simulink library "S2_aero_lib"  (Simulink 6.6)
libraries: simulink x1
settings Model: Creator=amurch  LastModifiedBy=Austin Murch

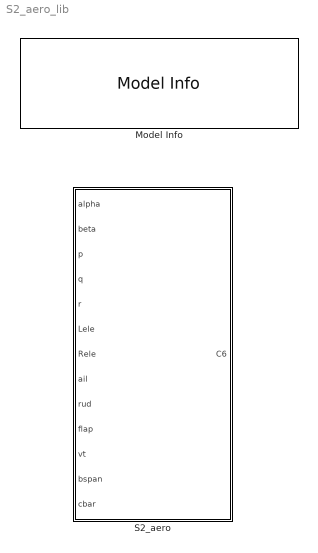
== system S2_aero_lib ==
  Model Info : simulink/Model-Wide Utilities/Model Info  SystemSampleTime=-1  InitialBlockCM=None  BlockCM=None  Frame=on  DisplayStringWithTags=|  HorizontalTextAlignment=Center  LeftAlignmentValue=0.5  SourceBlockDiagram=S2_aero_lib  TagMaxNumber=20
      | S2 Aerodynamic Model Library
      | %<ModelVersion>
      | Last modified by %<LastModifiedBy> on %<LastModificationDate>
  S2_aero : Stateflow chart

== matlab function S2_aero ==
  data: alpha input inherited; C6 output inherited; beta input inherited; p input inherited; q input inherited; r input inherited; Lele input inherited; Rele input inherited; ail input inherited; rud input inherited; flap input inherited; vt input inherited; bspan input inherited; cbar input inherited
function C6 =s2_aero(alpha,beta,p,q,r,Lele,Rele,ail,rud,flap,vt,bspan,cbar)
%
%  S2_AERO  Computes non-dimensional aerodynamic coefficients for the S2 aircraft.
%
%  Usage:
%  [C6]=s2_aero(alpha,beta,phat,qhat,rhat,throttle,ele,ail,rud,flap);
%
%  Description:
%
%    Computes the non-dimensional aerodynamic force and moment
%    coefficients for the S2 single-engine L-1011 model aircraft 
%    using frequency separation modeling and flight data from 
%    deployment 2007.02, September 2007.  
%
%
%  Input:
%    
%     alpha = angle of attack, deg.
%      beta = sideslip angle, deg.
%      phat = nondimensional roll rate (pb/2V), rad/sec.
%      qhat = nondimensional pitch rate (qc/2V), rad/sec.
%      rhat = nondimensional yaw rate (rb/2V), rad/sec.
%      Lele = left elevator deflection, deg.
%      Rele = right elevator deflection, deg.
%       ail = aileron deflection, deg.
%       rud = rudder deflection, deg.
%      flap = flap deflections, deg.
%        c = constants.
%            c.lim   = array of hard limits for the controls.

%  Output:
%
%     CX = body axis x force coefficient.
%     CY = body axis y force coefficient.
%     CZ = body axis z force coefficient.
%     C1 = rolling moment coefficient.
%     Cm = pitching moment coefficient.
%     Cn = yawing moment coefficient.
%

%
%    Calls:
%      s2_xo.m, s2_zo.m, s2_mo.m
%      s2_xd.m, s2_zd.m, s2_md.m
%      s2_yo.m, s2_1o.m, s2_no.m
%      s2_yd.m, s2_1d.m, s2_nd.m
%
%    Author:  Eugene A. Morelli
%
%    History:  
%      18 Feb 2008 - Created and debugged, EAM.
%      13 May 2008 - Modified for use in Simulink, AMM.
%
%  Copyright (C) 2008  Eugene A. Morelli
%
%  This program carries no warranty, not even the implied 
%  warranty of merchantability or fitness for a particular purpose.  
%
%  Please email bug reports or suggestions for improvements to:
%
%      e.a.morelli@nasa.gov
%
c.lim = [0 100;-30 30;-20 20;-30 30;0 30];
dtr=pi/180;
betar=beta*dtr;
alphar=alpha*dtr;
Lelr=Lele*dtr;
Relr=Rele*dtr;
elr = 0.5*(Lelr + Relr);
ailr=ail*dtr;
rdrr=rud*dtr;
flpr=flap*dtr;
phat = p*bspan/(2*vt);
qhat = q*cbar/(2*vt);
rhat = r*bspan/(2*vt);
ele_loc =10/12; % ft, location of center of elevator relative to butt line (approx)

%
%  Get the base terms.  
%
CXo=s2_xo(alphar,elr,flpr,c);
CZo=s2_zo(alphar,elr,flpr,c);
Cmo=s2_mo(alphar,elr,flpr,c);
%
CYo=s2_yo(alphar,elr,flpr,c);
C1o=s2_1o(alphar,elr,flpr,c);
Cno=s2_no(alphar,elr,flpr,c);
%
%  Get the stability and control derivatives. 
%
[CXa,CXq,CXel,CXflp]=s2_xd(alphar,elr,flpr,c);
[CZa,CZq,CZel,CZflp]=s2_zd(alphar,elr,flpr,c);
[Cma,Cmq,Cmel,Cmflp]=s2_md(alphar,elr,flpr,c);
%
[CYb,CYp,CYr,CYail,CYrdr]=s2_yd(alphar,elr,flpr,c);
[C1b,C1p,C1r,C1ail,C1rdr]=s2_1d(alphar,elr,flpr,c);
[Cnb,Cnp,Cnr,Cnail,Cnrdr]=s2_nd(alphar,elr,flpr,c);
%
%  Assemble the force and moment coefficients.
%
CX = CXo + CXq*qhat + CXflp*flpr + CXel*(Lelr + Relr)/2;
CZ = CZo + CZq*qhat + CZflp*flpr + CZel*(Lelr + Relr)/2;
Cm = Cmo + Cmq*qhat + Cmflp*flpr + Cmel*(Lelr + Relr)/2;
%
CY = CYo + CYb*betar + CYp*phat + CYr*rhat + CYail*ailr + CYrdr*rdrr;
C1 = C1o + C1b*betar + C1p*phat + C1r*rhat + C1ail*ailr + C1rdr*rdrr + CZel*ele_loc*(Relr - Lelr)/2/bspan;
Cn = Cno + Cnb*betar + Cnp*phat + Cnr*rhat + Cnail*ailr + Cnrdr*rdrr + CXel*ele_loc*(Lelr - Relr)/2/bspan;
%
% Apply some sanity limits to the coefficients
%
C6 = max(min([CX CY CZ C1 Cm Cn],[3 2 4 2 4 4]),-[3 2 4 2 4 4]);

function [CXo] = s2_xo(alpha,el,flp,c)
%
%  S2_XO  Computes the CX base aerodynamics.
%
%  Usage: CXo = s2_xo(alpha,el,flp,c);
%
%  Description:
%
%    Computes the CX base aerodynamics
%    for the S2 single-engine L-1011 model
%    aircraft nonlinear simulation.  
%
%  Input:
%    
%     alpha = angle of attack, rad.
%        el = elevator deflection, rad.
%       flp = flap deflection, rad.
%         c = c.c(1) through c.c(9) = inertia constants.
%  Output:
%
%       CXo = CX base aerodynamic term. 
%

%
%    Calls:
%      comfun.m
%
%    Author:  Eugene A. Morelli
%
%    History:  
%      05 May  2008 - Created and debugged, EAM.
%
%  Copyright (C) 2008  Eugene A. Morelli
%
%  This program carries no warranty, not even the implied 
%  warranty of merchantability or fitness for a particular purpose.  
%
%  Please email bug reports or suggestions for improvements to:
%
%      e.a.morelli@nasa.gov
%
dtr=pi/180;
x=[alpha,min(0,alpha-15*dtr)];
%
%  Cruise, flaps up, gear up, from flt9, man6.  
%
% IPXo=[0,1,11,10]';
% PXo=[ -0.080800885759421;...
%        0.820366736327515;...
%      -10.010727396895621;...
%        3.057073727021578];
% IPXo=[1,0,11,10]';
% PXo=[  0.822422596042795
%       -0.089099684117894
%      -11.674020983809706
%        3.480804446726977];
IPXo=[1,0,4,3]';
PXo=[  0.384250553871670;...
      -0.055695436673931;...
     -38.087897257727697;...
      14.888723078459181];
% IPXo=[0,1,2]';
% PXo=[ -0.070197931596795;...
%        0.703156250629286;...
%        0.250092538873889];
CXo=comfun(x,PXo,IPXo);
%
%  Approach, flaps down, gear down, from flt9, man9.
%
IPXoa=[0,1,2,11]';
PXoa=[ -0.341975568896875;...
        2.311938939310571;...
       -2.634264867496561;...
       -3.328376671167995];
CXoa=comfun(x,PXoa,IPXoa);
%
%  Compute df = fraction of full flap deflection.  
%
df=max(c.lim(5,1),min(flp/dtr,c.lim(5,2)))/c.lim(5,2);
%
%  Schedule linearly based on flap deflection.
%
CXo=CXo + df*(CXoa-CXo);
return


function [CXa,CXq,CXel,CXflp] = s2_xd(alpha,el,flp,c)
%
%  S2_XD  Computes the CX stability and control derivatives.
%
%  Usage: [CXa,CXq,CXel,CXflp] = s2_xd(alpha,el,flp,c);
%
%  Description:
%
%    Computes the CX stability and control derivatives 
%    for the S2 single-engine L-1011 model
%    aircraft nonlinear simulation.  
%
%  Input:
%    
%     alpha = angle of attack, rad.
%        el = elevator deflection, rad.
%       flp = flap deflection, rad.
%         c = c.c(1) through c.c(9) = inertia constants.
%  Output:
%
%       CXa = CX stability derivative for angle of attack, 1/rad.  
%       CXq = CX stability derivative for non-dimensional pitch rate.
%      CXel = CX control derivative for elevator deflection, 1/rad.
%     CXflp = CX control derivative for flap deflection, 1/rad.
%

%
%    Calls:
%      None
%
%    Author:  Eugene A. Morelli
%
%    History:  
%      05 May  2008 - Created and debugged, EAM.
%
%  Copyright (C) 2008  Eugene A. Morelli
%
%  This program carries no warranty, not even the implied 
%  warranty of merchantability or fitness for a particular purpose.  
%
%  Please email bug reports or suggestions for improvements to:
%
%      e.a.morelli@nasa.gov
%

%
%  Cruise, flaps up, gear up, from flt13, man8a.
%
CXa=0.4215;
CXq=0;
CXel=0.0375;
CXflp=0;
%
%  Approach, full flaps, gear down, from flt12, man6.
%
CXaa=0.4008;
CXqa=0;
CXela=0.0216;
CXflpa=0;
%
%  Compute df = fraction of full flap deflection.  
%
df=max(c.lim(5,1),min(flp*180/pi,c.lim(5,2)))/c.lim(5,2);
%
%  Schedule linearly based on flap deflection.
%
CXa=CXa + df*(CXaa-CXa);
CXq=CXq + df*(CXqa-CXq);
CXel=CXel + df*(CXela-CXel);
CXflp=CXflp + df*(CXflpa-CXflp);
return

function CYo = s2_yo(alpha,el,flp,c)
%
%  S2_YO  Computes the CY base aerodynamics.
%
%  Usage: CYo = s2_yo(alpha,el,flp,c);
%
%  Description:
%
%    Computes the CY base aerodynamics
%    for the S2 single-engine L-1011 model
%    aircraft nonlinear simulation.  
%
%  Input:
%    
%     alpha = angle of attack, rad.
%        el = elevator deflection, rad.
%       flp = flap deflection, rad.
%         c = c.c(1) through c.c(9) = inertia constants.
%  Output:
%
%       CYo = CY base aerodynamic term. 
%

%
%    Calls:
%      None
%
%    Author:  Eugene A. Morelli
%
%    History:  
%      05 May  2008 - Created and debugged, EAM.
%
%  Copyright (C) 2008  Eugene A. Morelli
%
%  This program carries no warranty, not even the implied 
%  warranty of merchantability or fitness for a particular purpose.  
%
%  Please email bug reports or suggestions for improvements to:
%
%      e.a.morelli@nasa.gov
%

CYo=0;
return

function [CYb,CYp,CYr,CYail,CYrdr] = s2_yd(alpha,el,flp,c)
%
%  S2_YD  Computes the CY stability and control derivatives.
%
%  Usage: [CYb,CYp,CYr,CYail,CYrdr] = s2_yd(alpha,el,flp,c);
%
%  Description:
%
%    Computes the CY stability and control derivatives 
%    for the S2 single-engine L-1011 model
%    aircraft nonlinear simulation.  
%
%  Input:
%    
%     alpha = angle of attack, rad.
%        el = elevator deflection, rad.
%       flp = flap deflection, rad.
%         c = c.c(1) through c.c(9) = inertia constants.
%             c.mass  = aircraft mass, slugs.
%             c.xcg   = longitudinal (MS) CG location, percent MAC.
%             c.ycg   = lateral (BL) CG location, in.
%             c.zcg   = vertical (WL) CG location, in.
%             c.xcgr  = reference longitudinal (MS) CG location, percent MAC.
%             c.heng  = angular momentum for rotating mass of the propulsion system.
%             c.sarea = wing reference area, ft2.
%             c.bspan = wing span, ft.
%             c.cbar  = wing MAC, ft.
%             c.lim   = array of hard limits for the controls.
%             c.ac    = name of the aircraft.
%             c.xfree = vector indicating free states for trim:
%                       = 1 for free state
%                       = 0 for fixed state
%             c.xinit = initial state vector for trim, 
%                       including fixed state values.
%             c.ufree = vector indicating free controls for trim:
%                       = 1 for free control
%                       = 0 for fixed control
%             c.uinit = initial control vector for trim, 
%                       including fixed control values.
%             c.gam   = flight path angle at trim, deg.
%             c.trate = turn rate at trim, deg/sec.
%             c.ltl   = trim or linearize flag
%                       =  1 for trim or steady condition
%                       =  0 for normal operation
%                       = -1 for linearization
%              c.ltrl = trim or linearize flag:
%                       = -1 for trim or steady condition
%                       =  0 for normal operation
%                       =  1 for linearization
%              c.lfi  = filter initialization flag:
%                       =  1 to initialize the filter
%                       =  0 for normal operation
%                       = -1 to skip the filtering (for numerical integration steps)
%              c.dt   = time step, sec.
%              c.x0   = initial state vector.
%              c.u0   = initial control vector.
%
%  Output:
%
%       CYb = CY stability derivative for angle of sideslip, 1/rad.  
%       CYp = CY stability derivative for non-dimensional roll rate.
%       CYr = CY stability derivative for non-dimensional yaw rate.
%     CYail = CY control derivative for aileron deflection, 1/rad.
%     CYrdr = CY control derivative for rudder deflection, 1/rad.
%

%
%    Calls:
%      None
%
%    Author:  Eugene A. Morelli
%
%    History:  
%      05 May  2008 - Created and debugged, EAM.
%
%  Copyright (C) 2008  Eugene A. Morelli
%
%  This program carries no warranty, not even the implied 
%  warranty of merchantability or fitness for a particular purpose.  
%
%  Please email bug reports or suggestions for improvements to:
%
%      e.a.morelli@nasa.gov
%

%
%  Cruise, flaps up, gear up, from flt13, man8a.
%
CYb=-0.7891;
CYp=0;
CYr=0;
CYail=0;
CYrdr=0.1881;
%
%  Approach, full flaps, gear down, from flt12, man6.
%
CYba=-1.0235;
CYpa=0;
CYra=0;
CYaila=0;
CYrdra=0.0835;
%
%  Compute df = fraction of full flap deflection.  
%
df=max(c.lim(5,1),min(flp*180/pi,c.lim(5,2)))/c.lim(5,2);
%
%  Schedule linearly based on flap deflection.
%
CYb=CYb + df*(CYba-CYb);
CYp=CYp + df*(CYpa-CYp);
CYr=CYr + df*(CYra-CYr);
CYail=CYail + df*(CYaila-CYail);
CYrdr=CYrdr + df*(CYrdra-CYrdr);
return


function CZo = s2_zo(alpha,el,flp,c)
%
%  S2_ZO  Computes the CZ base aerodynamics.
%
%  Usage: CZo = s2_zo(alpha,el,flp,c);
%
%  Description:
%
%    Computes the CZ base aerodynamics
%    for the S2 single-engine L-1011 model
%    aircraft nonlinear simulation.  
%
%  Input:
%    
%     alpha = angle of attack, rad.
%        el = elevator deflection, rad.
%       flp = flap deflection, rad.
%         c = c.c(1) through c.c(9) = inertia constants.
%             c.mass  = aircraft mass, slugs.
%             c.xcg   = longitudinal (MS) CG location, percent MAC.
%             c.ycg   = lateral (BL) CG location, in.
%             c.zcg   = vertical (WL) CG location, in.
%             c.xcgr  = reference longitudinal (MS) CG location, percent MAC.
%             c.heng  = angular momentum for rotating mass of the propulsion system.
%             c.sarea = wing reference area, ft2.
%             c.bspan = wing span, ft.
%             c.cbar  = wing MAC, ft.
%             c.lim   = array of hard limits for the controls.
%             c.ac    = name of the aircraft.
%             c.xfree = vector indicating free states for trim:
%                       = 1 for free state
%                       = 0 for fixed state
%             c.xinit = initial state vector for trim, 
%                       including fixed state values.
%             c.ufree = vector indicating free controls for trim:
%                       = 1 for free control
%                       = 0 for fixed control
%             c.uinit = initial control vector for trim, 
%                       including fixed control values.
%             c.gam   = flight path angle at trim, deg.
%             c.trate = turn rate at trim, deg/sec.
%             c.ltl   = trim or linearize flag
%                       =  1 for trim or steady condition
%                       =  0 for normal operation
%                       = -1 for linearization
%              c.ltrl = trim or linearize flag:
%                       = -1 for trim or steady condition
%                       =  0 for normal operation
%                       =  1 for linearization
%              c.lfi  = filter initialization flag:
%                       =  1 to initialize the filter
%                       =  0 for normal operation
%                       = -1 to skip the filtering (for numerical integration steps)
%              c.dt   = time step, sec.
%              c.x0   = initial state vector.
%              c.u0   = initial control vector.
%
%  Output:
%
%       CZo = CZ base aerodynamic term. 
%

%
%    Calls:
%      comfun.m
%
%    Author:  Eugene A. Morelli
%
%    History:  
%      05 May  2008 - Created and debugged, EAM.
%
%  Copyright (C) 2008  Eugene A. Morelli
%
%  This program carries no warranty, not even the implied 
%  warranty of merchantability or fitness for a particular purpose.  
%
%  Please email bug reports or suggestions for improvements to:
%
%      e.a.morelli@nasa.gov
%
dtr=pi/180;
x=[alpha,min(0,alpha-15*dtr)];
%
%  Cruise, flaps up, gear up, from flt9, man6.  
%
IPZo=[0,1,2]';
% PZo=[ -0.111682396118792;...
%       -3.997734371310473;...
%        3.374110079651810];
PZo=[ -0.094822381825331;...
      -4.321563667693882;...
       4.493418862269570];
% PZo=[ -2.093533523556459;...
%       0.991146827699140;...
%      -0.115181510304119];
% PZo=[-2.083281853665540;...
%       1.010713686289819;...
%      -0.112960033630600];
CZo=comfun(x,PZo,IPZo);
%
%  Approach, flaps down, gear down, from flt9, man9.
%
IPZoa=[0,1,11,2]';
PZoa=[ -0.283418187922199;...
       -3.886455168753432;...
        3.243978698447330;...
        2.311648275529938];
CZoa=comfun(x,PZoa,IPZoa);
%
%  Compute df = fraction of full flap deflection.  
%
df=max(c.lim(5,1),min(flp/dtr,c.lim(5,2)))/c.lim(5,2);
%
%  Schedule linearly based on flap deflection.
%
CZo=CZo + df*(CZoa-CZo);
return

function [CZa,CZq,CZel,CZflp] = s2_zd(alpha,el,flp,c)
%
%  S2_ZD  Computes the CZ stability and control derivatives.
%
%  Usage: [CZa,CZq,CZel,CZflp] = s2_zd(alpha,el,flp,c);
%
%  Description:
%
%    Computes the CZ stability and control derivatives 
%    for the S2 single-engine L-1011 model
%    aircraft nonlinear simulation.  
%
%  Input:
%    
%     alpha = angle of attack, rad.
%        el = elevator deflection, rad.
%       flp = flap deflection, rad.
%         c = c.c(1) through c.c(9) = inertia constants.
%             c.mass  = aircraft mass, slugs.
%             c.xcg   = longitudinal (MS) CG location, percent MAC.
%             c.ycg   = lateral (BL) CG location, in.
%             c.zcg   = vertical (WL) CG location, in.
%             c.xcgr  = reference longitudinal (MS) CG location, percent MAC.
%             c.heng  = angular momentum for rotating mass of the propulsion system.
%             c.sarea = wing reference area, ft2.
%             c.bspan = wing span, ft.
%             c.cbar  = wing MAC, ft.
%             c.lim   = array of hard limits for the controls.
%             c.ac    = name of the aircraft.
%             c.xfree = vector indicating free states for trim:
%                       = 1 for free state
%                       = 0 for fixed state
%             c.xinit = initial state vector for trim, 
%                       including fixed state values.
%             c.ufree = vector indicating free controls for trim:
%                       = 1 for free control
%                       = 0 for fixed control
%             c.uinit = initial control vector for trim, 
%                       including fixed control values.
%             c.gam   = flight path angle at trim, deg.
%             c.trate = turn rate at trim, deg/sec.
%             c.ltl   = trim or linearize flag
%                       =  1 for trim or steady condition
%                       =  0 for normal operation
%                       = -1 for linearization
%              c.ltrl = trim or linearize flag:
%                       = -1 for trim or steady condition
%                       =  0 for normal operation
%                       =  1 for linearization
%              c.lfi  = filter initialization flag:
%                       =  1 to initialize the filter
%                       =  0 for normal operation
%                       = -1 to skip the filtering (for numerical integration steps)
%              c.dt   = time step, sec.
%              c.x0   = initial state vector.
%              c.u0   = initial control vector.
%
%  Output:
%
%       CZa = CZ stability derivative for angle of attack, 1/rad.  
%       CZq = CZ stability derivative for non-dimensional pitch rate.
%      CZel = CZ control derivative for elevator deflection, 1/rad.
%     CZflp = CZ control derivative for flap deflection, 1/rad.
%

%
%    Calls:
%      None
%
%    Author:  Eugene A. Morelli
%
%    History:  
%      05 May  2008 - Created and debugged, EAM.
%
%  Copyright (C) 2008  Eugene A. Morelli
%
%  This program carries no warranty, not even the implied 
%  warranty of merchantability or fitness for a particular purpose.  
%
%  Please email bug reports or suggestions for improvements to:
%
%      e.a.morelli@nasa.gov
%

%
%  Cruise, flaps up, gear up, from flt13, man8a.
%
CZa=-4.286;
CZq=0;
CZel=-0.0396;
CZflp=0;
%
%  Approach, full flaps, gear down, from flt12, man6.
%
CZaa=-4.354;
CZqa=0;
CZela=-0.2233;
CZflpa=0;
%
%  Compute df = fraction of full flap deflection.  
%
df=max(c.lim(5,1),min(flp*180/pi,c.lim(5,2)))/c.lim(5,2);
%
%  Schedule linearly based on flap deflection.
%
CZa=CZa + df*(CZaa-CZa);
CZq=CZq + df*(CZqa-CZq);
CZel=CZel + df*(CZela-CZel);
CZflp=CZflp + df*(CZflpa-CZflp);
return

function C1o = s2_1o(alpha,el,flp,c)
%
%  S2_1O  Computes C1 base aerodynamics.
%
%  Usage: C1o = s2_1o(alpha,el,flp,c);
%
%  Description:
%
%    Computes C1 base aerodynamics
%    for the S2 single-engine L-1011 model
%    aircraft nonlinear simulation.  
%
%  Input:
%    
%     alpha = angle of attack, rad.
%        el = elevator deflection, rad.
%       flp = flap deflection, rad.
%         c = c.c(1) through c.c(9) = inertia constants.
%             c.mass  = aircraft mass, slugs.
%             c.xcg   = longitudinal (MS) CG location, percent MAC.
%             c.ycg   = lateral (BL) CG location, in.
%             c.zcg   = vertical (WL) CG location, in.
%             c.xcgr  = reference longitudinal (MS) CG location, percent MAC.
%             c.heng  = angular momentum for rotating mass of the propulsion system.
%             c.sarea = wing reference area, ft2.
%             c.bspan = wing span, ft.
%             c.cbar  = wing MAC, ft.
%             c.lim   = array of hard limits for the controls.
%             c.ac    = name of the aircraft.
%             c.xfree = vector indicating free states for trim:
%                       = 1 for free state
%                       = 0 for fixed state
%             c.xinit = initial state vector for trim, 
%                       including fixed state values.
%             c.ufree = vector indicating free controls for trim:
%                       = 1 for free control
%                       = 0 for fixed control
%             c.uinit = initial control vector for trim, 
%                       including fixed control values.
%             c.gam   = flight path angle at trim, deg.
%             c.trate = turn rate at trim, deg/sec.
%             c.ltl   = trim or linearize flag
%                       =  1 for trim or steady condition
%                       =  0 for normal operation
%                       = -1 for linearization
%              c.ltrl = trim or linearize flag:
%                       = -1 for trim or steady condition
%                       =  0 for normal operation
%                       =  1 for linearization
%              c.lfi  = filter initialization flag:
%                       =  1 to initialize the filter
%                       =  0 for normal operation
%                       = -1 to skip the filtering (for numerical integration steps)
%              c.dt   = time step, sec.
%              c.x0   = initial state vector.
%              c.u0   = initial control vector.
%
%  Output:
%
%       C1o = C1 base aerodynamic term. 
%

%
%    Calls:
%      None
%
%    Author:  Eugene A. Morelli
%
%    History:  
%      05 May  2008 - Created and debugged, EAM.
%
%  Copyright (C) 2008  Eugene A. Morelli
%
%  This program carries no warranty, not even the implied 
%  warranty of merchantability or fitness for a particular purpose.  
%
%  Please email bug reports or suggestions for improvements to:
%
%      e.a.morelli@nasa.gov
%

C1o=0;
return


function [C1b,C1p,C1r,C1ail,C1rdr] = s2_1d(alpha,el,flp,c)
%
%  S2_1D  Computes the C1 stability and control derivatives.
%
%  Usage: [C1b,C1p,C1r,C1ail,C1rdr] = s2_1d(alpha,el,flp,c);
%
%  Description:
%
%    Computes the C1 stability and control derivatives 
%    for the S2 single-engine L-1011 model
%    aircraft nonlinear simulation.  
%
%  Input:
%    
%     alpha = angle of attack, rad.
%        el = elevator deflection, rad.
%       flp = flap deflection, rad.
%         c = c.c(1) through c.c(9) = inertia constants.
%             c.mass  = aircraft mass, slugs.
%             c.xcg   = longitudinal (MS) CG location, percent MAC.
%             c.ycg   = lateral (BL) CG location, in.
%             c.zcg   = vertical (WL) CG location, in.
%             c.xcgr  = reference longitudinal (MS) CG location, percent MAC.
%             c.heng  = angular momentum for rotating mass of the propulsion system.
%             c.sarea = wing reference area, ft2.
%             c.bspan = wing span, ft.
%             c.cbar  = wing MAC, ft.
%             c.lim   = array of hard limits for the controls.
%             c.ac    = name of the aircraft.
%             c.xfree = vector indicating free states for trim:
%                       = 1 for free state
%                       = 0 for fixed state
%             c.xinit = initial state vector for trim, 
%                       including fixed state values.
%             c.ufree = vector indicating free controls for trim:
%                       = 1 for free control
%                       = 0 for fixed control
%             c.uinit = initial control vector for trim, 
%                       including fixed control values.
%             c.gam   = flight path angle at trim, deg.
%             c.trate = turn rate at trim, deg/sec.
%             c.ltl   = trim or linearize flag
%                       =  1 for trim or steady condition
%                       =  0 for normal operation
%                       = -1 for linearization
%              c.ltrl = trim or linearize flag:
%                       = -1 for trim or steady condition
%                       =  0 for normal operation
%                       =  1 for linearization
%              c.lfi  = filter initialization flag:
%                       =  1 to initialize the filter
%                       =  0 for normal operation
%                       = -1 to skip the filtering (for numerical integration steps)
%              c.dt   = time step, sec.
%              c.x0   = initial state vector.
%              c.u0   = initial control vector.
%
%  Output:
%
%       C1b = C1 stability derivative for angle of sideslip, 1/rad.  
%       C1p = C1 stability derivative for non-dimensional roll rate.
%       C1r = C1 stability derivative for non-dimensional yaw rate.
%     C1ail = C1 control derivative for aileron deflection, 1/rad.
%     C1rdr = C1 control derivative for rudder deflection, 1/rad.
%

%
%    Calls:
%      None
%
%    Author:  Eugene A. Morelli
%
%    History:  
%      05 May  2008 - Created and debugged, EAM.
%
%  Copyright (C) 2008  Eugene A. Morelli
%
%  This program carries no warranty, not even the implied 
%  warranty of merchantability or fitness for a particular purpose.  
%
%  Please email bug reports or suggestions for improvements to:
%
%      e.a.morelli@nasa.gov
%

%
%  Cruise, flaps up, gear up,from flt13, man8a.
%
C1b=-0.0874;
C1p=-0.3494;
C1r=0;
C1ail=-0.1106;
C1rdr=0.0222;
%
%  Approach, full flaps, gear down, from flt12, man6.
%
C1ba=-0.0999;
C1pa=-0.3370;
C1ra=0.2481;
C1aila=-0.1153;
C1rdra=0.0290;
%
%  Compute df = fraction of full flap deflection.  
%
df=max(c.lim(5,1),min(flp*180/pi,c.lim(5,2)))/c.lim(5,2);
%
%  Schedule linearly based on flap deflection.
%
C1b=C1b + df*(C1ba-C1b);
C1p=C1p + df*(C1pa-C1p);
C1r=C1r + df*(C1ra-C1r);
C1ail=C1ail + df*(C1aila-C1ail);
C1rdr=C1rdr + df*(C1rdra-C1rdr);
return

function Cmo = s2_mo(alpha,el,flp,c)
%
%  S2_MO  Computes the Cm base aerodynamics.
%
%  Usage: Cmo = s2_mo(alpha,el,flp,c);
%
%  Description:
%
%    Computes the Cm base aerodynamics
%    for the S2 single-engine L-1011 model
%    aircraft nonlinear simulation.  
%
%  Input:
%    
%     alpha = angle of attack, rad.
%        el = elevator deflection, rad.
%       flp = flap deflection, rad.
%         c = c.c(1) through c.c(9) = inertia constants.
%             c.mass  = aircraft mass, slugs.
%             c.xcg   = longitudinal (MS) CG location, percent MAC.
%             c.ycg   = lateral (BL) CG location, in.
%             c.zcg   = vertical (WL) CG location, in.
%             c.xcgr  = reference longitudinal (MS) CG location, percent MAC.
%             c.heng  = angular momentum for rotating mass of the propulsion system.
%             c.sarea = wing reference area, ft2.
%             c.bspan = wing span, ft.
%             c.cbar  = wing MAC, ft.
%             c.lim   = array of hard limits for the controls.
%             c.ac    = name of the aircraft.
%             c.xfree = vector indicating free states for trim:
%                       = 1 for free state
%                       = 0 for fixed state
%             c.xinit = initial state vector for trim, 
%                       including fixed state values.
%             c.ufree = vector indicating free controls for trim:
%                       = 1 for free control
%                       = 0 for fixed control
%             c.uinit = initial control vector for trim, 
%                       including fixed control values.
%             c.gam   = flight path angle at trim, deg.
%             c.trate = turn rate at trim, deg/sec.
%             c.ltl   = trim or linearize flag
%                       =  1 for trim or steady condition
%                       =  0 for normal operation
%                       = -1 for linearization
%              c.ltrl = trim or linearize flag:
%                       = -1 for trim or steady condition
%                       =  0 for normal operation
%                       =  1 for linearization
%              c.lfi  = filter initialization flag:
%                       =  1 to initialize the filter
%                       =  0 for normal operation
%                       = -1 to skip the filtering (for numerical integration steps)
%              c.dt   = time step, sec.
%              c.x0   = initial state vector.
%              c.u0   = initial control vector.
%
%  Output:
%
%       Cmo = Cm base aerodynamic term. 
%

%
%    Calls:
%      comfun.m
%
%    Author:  Eugene A. Morelli
%
%    History:  
%      05 May  2008 - Created and debugged, EAM.
%
%  Copyright (C) 2008  Eugene A. Morelli
%
%  This program carries no warranty, not even the implied 
%  warranty of merchantability or fitness for a particular purpose.  
%
%  Please email bug reports or suggestions for improvements to:
%
%      e.a.morelli@nasa.gov
%
dtr=pi/180;
x=[alpha,min(0,alpha-15*dtr)];
%
%  Cruise, flaps up, gear up, from flt9, man6.  
%
IPmo=[0,1,2,3]';
Pmo=[   0.115050347363051;...
       -3.747139267602230;...
       12.839049317550790;...
      -14.783755634585580];
% Pmo=[  0.090295231054901
%       -3.488208060494491
%       12.269780917782471
%      -15.073352650668282];
% IPmo=[1,0]';
% Pmo=[-0.075186283044130;...
%       0.016552669140252];
Cmo=comfun(x,Pmo,IPmo);
%
%  Approach, flaps down, gear down, from flt9, man9.
%
IPmoa=[1,0,2,3]';
Pmoa=[ -3.605802245160461
        0.189639137321186
       13.713160995340239
      -19.432849927441254];
Cmoa=comfun(x,Pmoa,IPmoa);
%
%  Compute df = fraction of full flap deflection.  
%
df=max(c.lim(5,1),min(flp/dtr,c.lim(5,2)))/c.lim(5,2);
%
%  Schedule linearly based on flap deflection.
%
Cmo=Cmo + df*(Cmoa-Cmo);
% %
% %  Stall model.
% %
% IPmos=[0,10,100]';
% Pmos=[ -0.304253041325711;...
%        -1.344781926737646;...
%       -50.714930712751745];
% Cmos=comfun(x,Pmos,IPmos);
% %
% %  Blend the stall model to avoid discontinuities.
% %
% %  Mean values and standard deviations 
% %  for the longitudinal angle of attack subspace 
% %  transition region.  
% %
% abar=[13,17]*dtr;
% asig=[ 2, 2]*dtr;
% % if alpha > abar(1,2)-4*asig(1,2) & alpha < abar(1,1)+4*asig(1,1)
% %   gw1=gauss(alpha,abar(1,1),asig(1,1)^2,1);
% %   gw2=gauss(alpha,abar(1,2),asig(1,2)^2,1);
% %   w1=gw1/(gw1+gw2);
% %   w2=gw2/(gw1+gw2);
% %   Cmo=w1*Cmo+w2*Cmos;
% % elseif alpha >= abar(1,1)+4*asig(1,1)
% %   Cmo=Cmos;
% % end
return


function [Cma,Cmq,Cmel,Cmflp] = s2_md(alpha,el,flp,c)
%
%  S2_MD  Computes the Cm stability and control derivatives.
%
%  Usage: [Cma,Cmq,Cmel,Cmflp] = s2_md(alpha,el,flp,c);
%
%  Description:
%
%    Computes the Cm stability and control derivatives 
%    for the S2 single-engine L-1011 model
%    aircraft nonlinear simulation.  
%
%  Input:
%    
%     alpha = angle of attack, rad.
%        el = elevator deflection, rad.
%       flp = flap deflection, rad.
%         c = c.c(1) through c.c(9) = inertia constants.
%             c.mass  = aircraft mass, slugs.
%             c.xcg   = longitudinal (MS) CG location, percent MAC.
%             c.ycg   = lateral (BL) CG location, in.
%             c.zcg   = vertical (WL) CG location, in.
%             c.xcgr  = reference longitudinal (MS) CG location, percent MAC.
%             c.heng  = angular momentum for rotating mass of the propulsion system.
%             c.sarea = wing reference area, ft2.
%             c.bspan = wing span, ft.
%             c.cbar  = wing MAC, ft.
%             c.lim   = array of hard limits for the controls.
%             c.ac    = name of the aircraft.
%             c.xfree = vector indicating free states for trim:
%                       = 1 for free state
%                       = 0 for fixed state
%             c.xinit = initial state vector for trim, 
%                       including fixed state values.
%             c.ufree = vector indicating free controls for trim:
%                       = 1 for free control
%                       = 0 for fixed control
%             c.uinit = initial control vector for trim, 
%                       including fixed control values.
%             c.gam   = flight path angle at trim, deg.
%             c.trate = turn rate at trim, deg/sec.
%             c.ltl   = trim or linearize flag
%                       =  1 for trim or steady condition
%                       =  0 for normal operation
%                       = -1 for linearization
%              c.ltrl = trim or linearize flag:
%                       = -1 for trim or steady condition
%                       =  0 for normal operation
%                       =  1 for linearization
%              c.lfi  = filter initialization flag:
%                       =  1 to initialize the filter
%                       =  0 for normal operation
%                       = -1 to skip the filtering (for numerical integration steps)
%              c.dt   = time step, sec.
%              c.x0   = initial state vector.
%              c.u0   = initial control vector.
%
%  Output:
%
%       Cma = Cm stability derivative for angle of attack, 1/rad.  
%       Cmq = Cm stability derivative for non-dimensional pitch rate.
%      Cmel = Cm control derivative for elevator deflection, 1/rad.
%     Cmflp = Cm control derivative for flap deflection, 1/rad.
%

%
%    Calls:
%      None
%
%    Author:  Eugene A. Morelli
%
%    History:  
%      05 May  2008 - Created and debugged, EAM.
%
%  Copyright (C) 2008  Eugene A. Morelli
%
%  This program carries no warranty, not even the implied 
%  warranty of merchantability or fitness for a particular purpose.  
%
%  Please email bug reports or suggestions for improvements to:
%
%      e.a.morelli@nasa.gov
%

%
%  Cruise, flaps up, gear up, from flt13, man8a.
%
Cma=-1.355;
Cmq=-26.01;
Cmel=-1.069;
Cmflp=0;
%
%  Approach, full flaps, gear down, from flt12, man6.
%
Cmaa=-1.490;
Cmqa=-23.21;
Cmela=-1.112;
Cmflpa=0;
%
%  Compute df = fraction of full flap deflection.  
%
df=max(c.lim(5,1),min(flp*180/pi,c.lim(5,2)))/c.lim(5,2);
%
%  Schedule linearly based on flap deflection.
%
Cma=Cma + df*(Cmaa-Cma);
Cmq=Cmq + df*(Cmqa-Cmq);
Cmel=Cmel + df*(Cmela-Cmel);
Cmflp=Cmflp + df*(Cmflpa-Cmflp);
return


function Cno = s2_no(alpha,el,flp,c)
%
%  S2_NO  Computes the Cn base aerodynamics.
%
%  Usage: Cno = s2_no(alpha,el,flp,c);
%
%  Description:
%
%    Computes the Cn base aerodynamics
%    for the S2 single-engine L-1011 model
%    aircraft nonlinear simulation.  
%
%  Input:
%    
%     alpha = angle of attack, rad.
%        el = elevator deflection, rad.
%       flp = flap deflection, rad.
%         c = c.c(1) through c.c(9) = inertia constants.
%             c.mass  = aircraft mass, slugs.
%             c.xcg   = longitudinal (MS) CG location, percent MAC.
%             c.ycg   = lateral (BL) CG location, in.
%             c.zcg   = vertical (WL) CG location, in.
%             c.xcgr  = reference longitudinal (MS) CG location, percent MAC.
%             c.heng  = angular momentum for rotating mass of the propulsion system.
%             c.sarea = wing reference area, ft2.
%             c.bspan = wing span, ft.
%             c.cbar  = wing MAC, ft.
%             c.lim   = array of hard limits for the controls.
%             c.ac    = name of the aircraft.
%             c.xfree = vector indicating free states for trim:
%                       = 1 for free state
%                       = 0 for fixed state
%             c.xinit = initial state vector for trim, 
%                       including fixed state values.
%             c.ufree = vector indicating free controls for trim:
%                       = 1 for free control
%                       = 0 for fixed control
%             c.uinit = initial control vector for trim, 
%                       including fixed control values.
%             c.gam   = flight path angle at trim, deg.
%             c.trate = turn rate at trim, deg/sec.
%             c.ltl   = trim or linearize flag
%                       =  1 for trim or steady condition
%                       =  0 for normal operation
%                       = -1 for linearization
%              c.ltrl = trim or linearize flag:
%                       = -1 for trim or steady condition
%                       =  0 for normal operation
%                       =  1 for linearization
%              c.lfi  = filter initialization flag:
%                       =  1 to initialize the filter
%                       =  0 for normal operation
%                       = -1 to skip the filtering (for numerical integration steps)
%              c.dt   = time step, sec.
%              c.x0   = initial state vector.
%              c.u0   = initial control vector.
%
%  Output:
%
%       Cno = Cn base aerodynamic term. 
%

%
%    Calls:
%      None
%
%    Author:  Eugene A. Morelli
%
%    History:  
%      05 May  2008 - Created and debugged, EAM.
%
%  Copyright (C) 2008  Eugene A. Morelli
%
%  This program carries no warranty, not even the implied 
%  warranty of merchantability or fitness for a particular purpose.  
%
%  Please email bug reports or suggestions for improvements to:
%
%      e.a.morelli@nasa.gov
%

Cno=0;
return


function [Cnb,Cnp,Cnr,Cnail,Cnrdr] = s2_nd(alpha,el,flp,c)
%
%  S2_ND  Computes the Cn stability and control derivatives.
%
%  Usage: [Cnb,Cnp,Cnr,Cnail,Cnrdr] = s2_nd(alpha,el,flp,c);
%
%  Description:
%
%    Computes the Cn stability and control derivatives 
%    for the S2 single-engine L-1011 model
%    aircraft nonlinear simulation.  
%
%  Input:
%    
%     alpha = angle of attack, rad.
%        el = elevator deflection, rad.
%       flp = flap deflection, rad.
%         c = c.c(1) through c.c(9) = inertia constants.
%             c.mass  = aircraft mass, slugs.
%             c.xcg   = longitudinal (MS) CG location, percent MAC.
%             c.ycg   = lateral (BL) CG location, in.
%             c.zcg   = vertical (WL) CG location, in.
%             c.xcgr  = reference longitudinal (MS) CG location, percent MAC.
%             c.heng  = angular momentum for rotating mass of the propulsion system.
%             c.sarea = wing reference area, ft2.
%             c.bspan = wing span, ft.
%             c.cbar  = wing MAC, ft.
%             c.lim   = array of hard limits for the controls.
%             c.ac    = name of the aircraft.
%             c.xfree = vector indicating free states for trim:
%                       = 1 for free state
%                       = 0 for fixed state
%             c.xinit = initial state vector for trim, 
%                       including fixed state values.
%             c.ufree = vector indicating free controls for trim:
%                       = 1 for free control
%                       = 0 for fixed control
%             c.uinit = initial control vector for trim, 
%                       including fixed control values.
%             c.gam   = flight path angle at trim, deg.
%             c.trate = turn rate at trim, deg/sec.
%             c.ltl   = trim or linearize flag
%                       =  1 for trim or steady condition
%                       =  0 for normal operation
%                       = -1 for linearization
%              c.ltrl = trim or linearize flag:
%                       = -1 for trim or steady condition
%                       =  0 for normal operation
%                       =  1 for linearization
%              c.lfi  = filter initialization flag:
%                       =  1 to initialize the filter
%                       =  0 for normal operation
%                       = -1 to skip the filtering (for numerical integration steps)
%              c.dt   = time step, sec.
%              c.x0   = initial state vector.
%              c.u0   = initial control vector.
%
%  Output:
%
%       Cnb = Cn stability derivative for angle of sideslip, 1/rad.  
%       Cnp = Cn stability derivative for non-dimensional roll rate.
%       Cnr = Cn stability derivative for non-dimensional yaw rate.
%     Cnail = Cn control derivative for aileron deflection, 1/rad.
%     Cnrdr = Cn control derivative for rudder deflection, 1/rad.
%

%
%    Calls:
%      None
%
%    Author:  Eugene A. Morelli
%
%    History:  
%      05 May  2008 - Created and debugged, EAM.
%
%  Copyright (C) 2008  Eugene A. Morelli
%
%  This program carries no warranty, not even the implied 
%  warranty of merchantability or fitness for a particular purpose.  
%
%  Please email bug reports or suggestions for improvements to:
%
%      e.a.morelli@nasa.gov
%

%
%  Cruise, flaps up, gear up, from flt13, man8a.
%
Cnb=0.1334;
Cnp=0;
Cnr=-0.3323;
Cnail=0.0153;
Cnrdr=-0.0805;
%
%  Approach, full flaps, gear down, from flt12, man6.
%
Cnba=0.1533;
Cnpa=0;
Cnra=-0.2846;
Cnaila=0.0177;
Cnrdra=-0.0765;
%
%  Compute df = fraction of full flap deflection.  
%
df=max(c.lim(5,1),min(flp*180/pi,c.lim(5,2)))/c.lim(5,2);
%
%  Schedule linearly based on flap deflection.
%
Cnb=Cnb + df*(Cnba-Cnb);
Cnp=Cnp + df*(Cnpa-Cnp);
Cnr=Cnr + df*(Cnra-Cnr);
Cnail=Cnail + df*(Cnaila-Cnail);
Cnrdr=Cnrdr + df*(Cnrdra-Cnrdr);
return


function [y,xp] = comfun(x,ap,iap)
%
%  COMFUN  Computes the value of ordinary polynomial functions.  
%
%  Usage: [y,xp] = comfun(x,ap,iap);
%
%  Description:
%
%    Computes the function y as an ordinary polynomial expansion 
%    with length(iap) terms.  Vector iap specifies the powers of the 
%    independent variables contained in columns of x, and vector ap 
%    contains the parameter values.  The powers of the
%    independent variables contained in each element of vector iap
%    from least significant digit to most significant digit 
%    correspond to the columns of matrix x in order.  
%
%  Input:
%    
%      x = matrix of independent variable vectors.
%     ap = vector of parameter values for each polynomial term.
%    iap = vector of integers indicating powers of the independent 
%          variables for each polynomial term.
%
%  Output:
%
%      y = polynomial function of the independent variables in x.
%     xp = matrix of independent variable functions generated
%          from x according to iap.  
%

%
%    Calls:
%      cvec.m
%
%    Author:  Eugene A. Morelli
%
%    History:  
%      14 Nov 1995 - Created and debugged, EAM.
%      10 Dec 2000 - Vectorized and changed input/output, EAM.
%
%  Copyright (C) 2006  Eugene A. Morelli
%
%  This program carries no warranty, not even the implied 
%  warranty of merchantability or fitness for a particular purpose.  
%
%  Please email bug reports or suggestions for improvements to:
%
%      e.a.morelli@nasa.gov
%
[npts,nvar]=size(x);
nterms=length(iap);
ap=cvec(ap);
%
%  Generate the polynomial function matrix and the final model
%  output based on the polynomial functions.
%
xp=ones(npts,nterms);
for i=1:nterms,
  indx=iap(i);
  for j=1:nvar,
    ji=round(rem(indx,10));
    if ji~=0
      xp(:,i)=xp(:,i).*(x(:,j).^ji);
    end
    indx=floor(indx/10);
  end
end
%
%  Compute the model output.
%
y=xp*ap(1:nterms);
return


function yc = cvec(y)
%
%  CVEC  Makes any input vector into a column vector.  
%
%  Usage: yc = cvec(y);
%
%  Description:
%
%    Makes y vector into a column vector. 
%
%  Input:
%    
%    y = input vector.
%
%  Output:
%
%    yc = column vector with same elements as y.
%

%
%    Calls:
%      None
%
%    Author:  Eugene A. Morelli
%
%    History:  
%      02 Mar 2000 - Created and debugged, EAM.
%
%  Copyright (C) 2006  Eugene A. Morelli
%
%  This program carries no warranty, not even the implied 
%  warranty of merchantability or fitness for a particular purpose.  
%
%  Please email bug reports or suggestions for improvements to:
%
%      e.a.morelli@nasa.gov
%
[m,n]=size(y);
if n > m
  yc=y';
else
  yc=y;
end
yc=yc(:,1);
return
